simulink model "launch_controller"  (R2024b)
settings: Solver=FixedStepAuto  StartTime=0.0  StopTime=10.0  FixedStep=0.004  RelTol=1e-3
settings Model: Creator=lukec  LastModifiedBy=lukec
settings OptimizationCC: DefaultParameterBehavior=Inlined  EnhancedBackFolding=on  PassReuseOutputArgsAs=Individual arguments  ZeroExternalMemoryAtStartup=off  ZeroInternalMemoryAtStartup=off  OptimizeBlockOrder=speed  DifferentSizesBufferReuse=on  OptimizationCustomize=off  EfficientTunableParamExpr=on
settings DebuggingCC: ParameterTunabilityLossMsg=error
settings SFSimCC: MATLABDynamicMemAlloc=off
settings RTWCC: Description=Embedded Coder  SystemTargetFile=ert.tlc  GenCodeOnly=on  PackageGeneratedCodeAndArtifacts=on  TemplateMakefile=ert_default_tmf  Toolchain=CMake  TargetLang=C++
settings CodeAppCC: ForceParamTrailComments=on  IgnoreCustomStorageClasses=off  MaxIdLength=128  OperatorAnnotations=on  SimulinkDataObjDesc=on  SFDataObjDesc=on  InsertBlockDesc=on
settings ERTTargetCC: TargetLangStandard=C++11 (ISO)  GenerateSampleERTMain=on  CodeInterfacePackaging=C++ class  RootIOFormat=Structure reference  ERTCustomFileTemplate=example_file_process.tlc

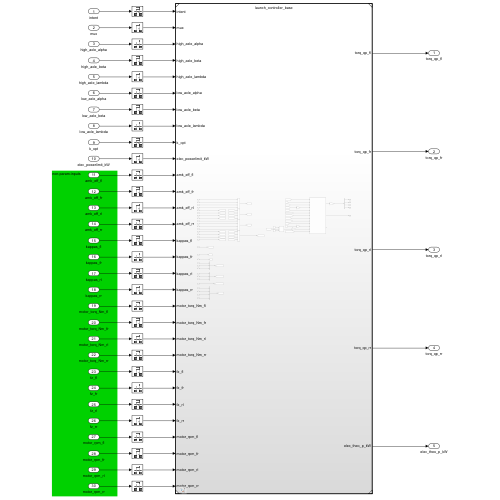
[thumbnail: Simulink's stored preview of the top-level diagram]
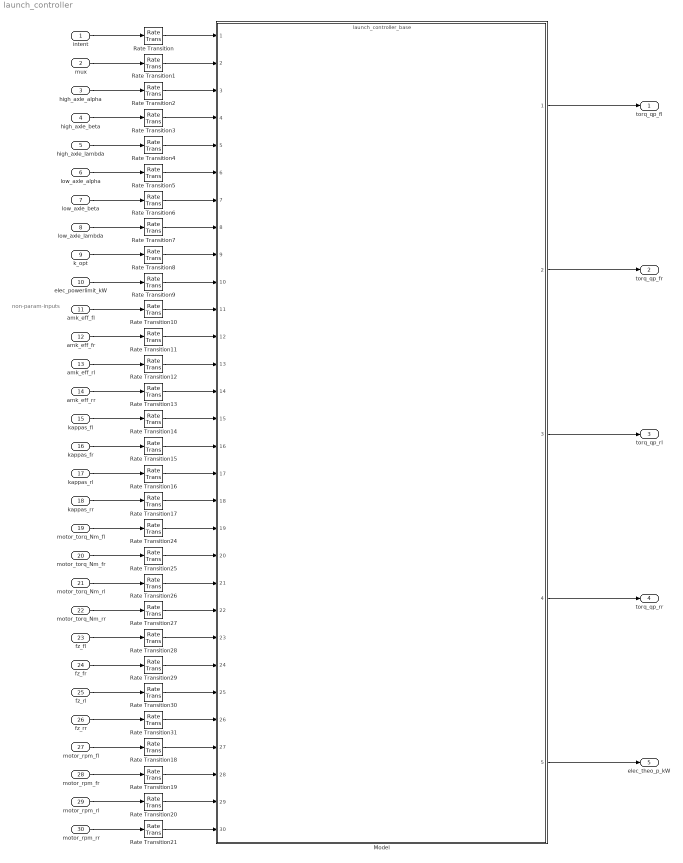
== system launch_controller ==
  note: non-param-inputs
  intent : Inport
  mux : Inport  Port=2
  high_axle_alpha : Inport  Port=3
  high_axle_beta : Inport  Port=4
  high_axle_lambda : Inport  Port=5
  low_axle_alpha : Inport  Port=6
  low_axle_beta : Inport  Port=7
  low_axle_lambda : Inport  Port=8
  k_opt : Inport  Port=9
  elec_powerlimit_kW : Inport  Port=10
  amk_eff_fl : Inport  Port=11
  amk_eff_fr : Inport  Port=12
  amk_eff_rl : Inport  Port=13
  amk_eff_rr : Inport  Port=14
  kappas_fl : Inport  Port=15
  kappas_fr : Inport  Port=16
  kappas_rl : Inport  Port=17
  kappas_rr : Inport  Port=18
  motor_torq_Nm_fl : Inport  Port=19
  motor_torq_Nm_fr : Inport  Port=20
  motor_torq_Nm_rl : Inport  Port=21
  motor_torq_Nm_rr : Inport  Port=22
  fz_fl : Inport  Port=23
  fz_fr : Inport  Port=24
  fz_rl : Inport  Port=25
  fz_rr : Inport  Port=26
  motor_rpm_fl : Inport  Port=27
  motor_rpm_fr : Inport  Port=28
  motor_rpm_rl : Inport  Port=29
  motor_rpm_rr : Inport  Port=30
  Model : ModelReference  ModelNameDialog=launch_controller_base.slx  SimulationMode=Normal  ModelReferenceVersion=1.5
  Rate Transition{,1..21,24..31} (30 alike) : RateTransition  OutPortSampleTime=0.004
  torq_qp_fl : Outport
  torq_qp_fr : Outport  Port=2
  torq_qp_rl : Outport  Port=3
  torq_qp_rr : Outport  Port=4
  elec_theo_p_kW : Outport  Port=5
  wires:
  Rate Transition16/1 -> Model/17
  Rate Transition30/1 -> Model/25
  Rate Transition27/1 -> Model/22
  Rate Transition28/1 -> Model/23
  Rate Transition26/1 -> Model/21
  Rate Transition21/1 -> Model/30
  Rate Transition31/1 -> Model/26
  Rate Transition25/1 -> Model/20
  Rate Transition18/1 -> Model/27
  Rate Transition/1 -> Model/1
  Rate Transition24/1 -> Model/19
  fz_rl/1 -> Rate Transition30/1
  fz_fr/1 -> Rate Transition29/1
  Rate Transition3/1 -> Model/4
  Rate Transition2/1 -> Model/3
  motor_rpm_rr/1 -> Rate Transition21/1
  k_opt/1 -> Rate Transition8/1
  Rate Transition17/1 -> Model/18
  Rate Transition1/1 -> Model/2
  kappas_fr/1 -> Rate Transition15/1
  amk_eff_fl/1 -> Rate Transition10/1
  Rate Transition7/1 -> Model/8
  fz_rr/1 -> Rate Transition31/1
  amk_eff_rl/1 -> Rate Transition12/1
  Rate Transition5/1 -> Model/6
  motor_torq_Nm_rl/1 -> Rate Transition26/1
  high_axle_beta/1 -> Rate Transition3/1
  motor_rpm_rl/1 -> Rate Transition20/1
  Rate Transition14/1 -> Model/15
  low_axle_beta/1 -> Rate Transition6/1
  Rate Transition9/1 -> Model/10
  Rate Transition4/1 -> Model/5
  Rate Transition12/1 -> Model/13
  kappas_rl/1 -> Rate Transition16/1
  Rate Transition15/1 -> Model/16
  Rate Transition13/1 -> Model/14
  Rate Transition11/1 -> Model/12
  kappas_fl/1 -> Rate Transition14/1
  Rate Transition10/1 -> Model/11
  motor_rpm_fl/1 -> Rate Transition18/1
  motor_rpm_fr/1 -> Rate Transition19/1
  low_axle_alpha/1 -> Rate Transition5/1
  high_axle_alpha/1 -> Rate Transition2/1
  Rate Transition8/1 -> Model/9
  Rate Transition20/1 -> Model/29
  kappas_rr/1 -> Rate Transition17/1
  Rate Transition19/1 -> Model/28
  intent/1 -> Rate Transition/1
  motor_torq_Nm_fl/1 -> Rate Transition24/1
  high_axle_lambda/1 -> Rate Transition4/1
  mux/1 -> Rate Transition1/1
  motor_torq_Nm_fr/1 -> Rate Transition25/1
  Rate Transition6/1 -> Model/7
  Rate Transition29/1 -> Model/24
  elec_powerlimit_kW/1 -> Rate Transition9/1
  amk_eff_rr/1 -> Rate Transition13/1
  amk_eff_fr/1 -> Rate Transition11/1
  low_axle_lambda/1 -> Rate Transition7/1
  motor_torq_Nm_rr/1 -> Rate Transition27/1
  fz_fl/1 -> Rate Transition28/1
  Model/1 -> torq_qp_fl/1
  Model/2 -> torq_qp_fr/1
  Model/3 -> torq_qp_rl/1
  Model/4 -> torq_qp_rr/1
  Model/5 -> elec_theo_p_kW/1
